simulink model "compensacion_analogica_integrador"  (R2014b)
settings: Solver=ode45  StartTime=0.0  StopTime=4  RelTol=1e-3  EnableMultiTasking=on
settings Model: Creator=Javi  LastModifiedBy=Javi
settings OptimizationCC: UseDivisionForNetSlopeComputation=off  SimCompilerOptimization=off
settings DebuggingCC: FcnCallInpInsideContextMsg=error  FrameProcessingCompatibilityMsg=error  SFExecutionAtInitializationDiag=none
settings HardwareCC: ProdBitPerSizeT=32  ProdBitPerPtrDiffT=32
settings RTWCC: RTWCompilerOptimization=off
settings ConfigComp: CovMetricSettings=dw  CovHtmlReporting=on  CovSaveCumulativeToWorkspaceVar=on  CovSaveSingleToWorkspaceVar=on  CovExternalEMLEnable=off  CovSFcnEnable=off

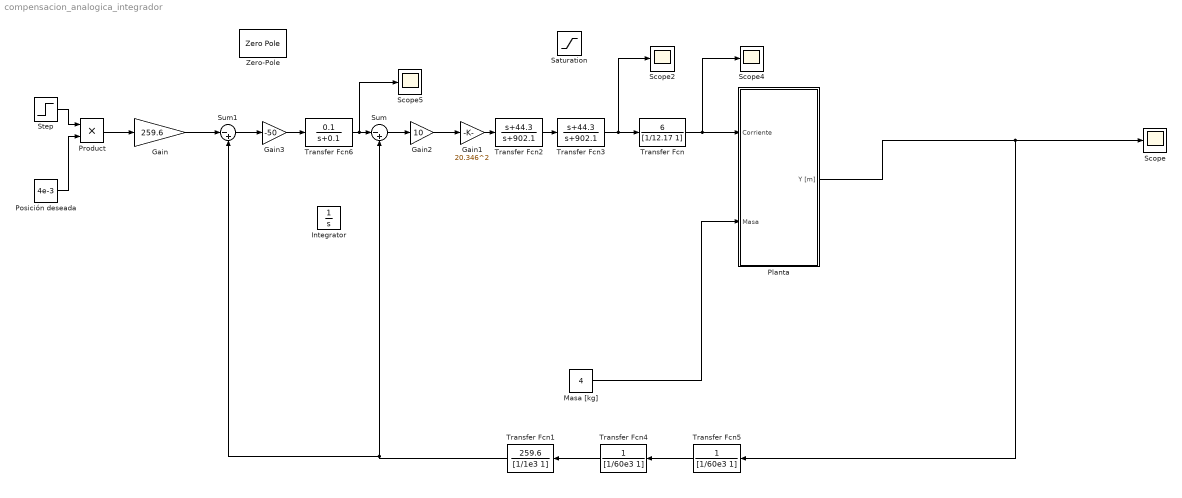
== system compensacion_analogica_integrador ==
  Gain : Gain  Gain=259.6
  Gain1 : Gain  Gain=20.346^2
  Gain2 : Gain  Gain=10
  Gain3 : Gain  Gain=-50
  Integrator : Integrator
  "Masa [kg] " : Constant  Value=4
  "Planta " : Subsystem
  Posición deseada : Constant  Value=4e-3
  Product : Product
  Saturation : Saturate  UpperLimit=5  LowerLimit=-inf
  Scope{,2,4..5} (4 alike) : Scope
      Scope settings: TimeRange=4  YMin=0  YMax=0.014
      Scope2 settings: TimeRange=0.005185185185185187  YMin=-3500000  YMax=500000  SaveName=ScopeData2
      Scope4 settings: TimeRange=0.005185185185185187  YMin=-3500000  YMax=500000  SaveName=ScopeData4
      Scope5 settings: TimeRange=4  YMin=-0.1  YMax=0.9  SaveName=ScopeData5
  Step : Step  Time=0.01  SampleTime=0
  Sum : Sum  Inputs=|-+
  Sum1 : Sum  Inputs=|-+
  Transfer Fcn : TransferFcn  Numerator=[6]  Denominator=[1/12.17 1]
  Transfer Fcn1 : TransferFcn  Numerator=259.6  Denominator=[1/1e3 1]
  Transfer Fcn2 : TransferFcn  Numerator=[1 44.3]  Denominator=[1 902.1]
  Transfer Fcn3 : TransferFcn  Numerator=[1 44.3]  Denominator=[1 902.1]
  Transfer Fcn4 : TransferFcn  Numerator=1  Denominator=[1/60e3 1]
  Transfer Fcn5 : TransferFcn  Numerator=1  Denominator=[1/60e3 1]
  Transfer Fcn6 : TransferFcn  Numerator=[0.1]  Denominator=[1 0.1]
  Zero-Pole : ZeroPole  Zeros=[-221.7 -221.7]  Poles=[-4511 -4511]  Gain=8.28e5
  wires:
  "Masa [kg] "/1 -> "Planta "/2("Masa ")
  "Planta "/1(Y [m]) -> Transfer Fcn5/1, Scope/1
  Transfer Fcn1/1 -> Sum1/2, Sum/2
  Transfer Fcn/1 -> "Planta "/1(Corriente), Scope4/1
  Transfer Fcn3/1 -> Scope2/1, Transfer Fcn/1
  Step/1 -> Product/1
  Posición deseada/1 -> Product/2
  Product/1 -> Gain/1
  Transfer Fcn2/1 -> Transfer Fcn3/1
  Gain1/1 -> Transfer Fcn2/1
  Sum/1 -> Gain2/1
  Gain2/1 -> Gain1/1
  Transfer Fcn4/1 -> Transfer Fcn1/1
  Transfer Fcn5/1 -> Transfer Fcn4/1
  Gain/1 -> Sum1/1
  Sum1/1 -> Gain3/1
  Gain3/1 -> Transfer Fcn6/1
  Transfer Fcn6/1 -> Scope5/1, Sum/1

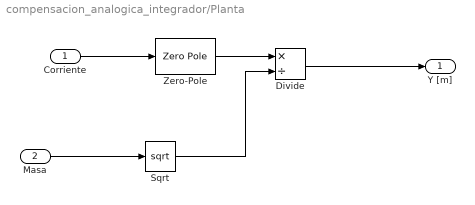
== system compensacion_analogica_integrador/Planta  ==
  Corriente : Inport
  "Masa " : Inport  Port=2
  Divide : Product  Inputs=*/
  Sqrt : Sqrt  SaturateOnIntegerOverflow=on
  Zero-Pole : ZeroPole  Zeros=[]  Poles=[70 -70]  Gain=-6.58
  Y [m] : Outport
  wires:
  Divide/1 -> Y [m]/1
  Corriente/1 -> Zero-Pole/1
  Zero-Pole/1 -> Divide/1
  "Masa "/1 -> Sqrt/1
  Sqrt/1 -> Divide/2
